simulink model "Cmd_vectorielle_simscape_tri5"  (R2018b)
settings: Solver=ode4  StartTime=0.0  StopTime=Tsim_all  FixedStep=Ts  RelTol=1e-4
values from neighbouring files (symbols this model uses):
  Clarke = [2/3 -1/3 -1/3;0 1/sqrt(3) -1/sqrt(3);1/3 1/3 1/3]    [Init_MS.m]
  Cn = Pn*rendn/Wn    (= 4.58366236105)    [Init_MS.m]
  delay_torque = 15    [Init_MS.m]
  fv = 0.0033    [Init_MS.m]
  IClarke = [1 0 1;-1/2 sqrt(3)/2 1;-1/2 -sqrt(3)/2 1]    [Init_MS.m]
  Idref = 0    [Init_MS.m]
  J = 0.05    [Init_MS.m]
  kc = 3/2*p*Phi_f    (= 2.133)    [Init_MS.m]
  Kpd_simscape = n*Rs    (= 42)    [Init_MS.m]
  Kpq_simscape = n*Rs    (= 42)    [Init_MS.m]
  kv = 5*fv/kc    (= 0.00773558368495)    [Init_MS.m]
  Ld = 0.245    [Init_MS.m]
  Lq = Ld    (= 0.245)    [Init_MS.m]
  p = 2    [Init_MS.m]
  Phi_f = 0.711    [Init_MS.m]
  r = 0.8    [Init_MS.m]
  Rs = 10.5    [Init_MS.m]
  Tid = Ld/Rs    (= 0.0233333333333)    [Init_MS.m]
  Tiq = Lq/Rs    (= 0.0233333333333)    [Init_MS.m]
  Ts = 1e-5    (= 1e-05)    [Init_MS.m]
  Vdc = 550    [Init_MS.m]
  Vn = 220    [Init_MS.m]
  Wn = Nn*2*pi/60    (= 157.079632679)    [Init_MS.m]
libraries: powerlib x5, powerlib_meascontrol x1
Description:
  | Copyright 2008-2020 The MathWorks, Inc.
settings Model: ExtModeTrigMode=oneshot  ExtModeArmWhenConnect=off  ExtModeAutoUpdateStatusClock=off  Creator=MathWorks  LastModifiedBy=jras
settings SolverCC: ZeroCrossAlgorithm=Adaptive
settings DataIOCC: ExternalInput=[]  SaveFormat=Array  SignalLoggingSaveFormat=ModelDataLogs  SaveOutput=off  SignalLogging=off  DSMLogging=off  SaveTime=off  SignalLoggingName=sigsOut
settings OptimizationCC: BlockReduction=off  BooleanDataType=off  ExpressionDepthLimit=2147483647  InitFltsAndDblsToZero=on  EfficientMapNaN2IntZero=off  LifeSpan=inf
settings DebuggingCC: UnderspecifiedInitializationDetection=Classic  MergeDetectMultiDrivingBlocksExec=none  CheckExecutionContextPreStartOutputMsg=on  CheckExecutionContextRuntimeOutputMsg=on  SignalResolutionControl=TryResolveAllWithWarning  IgnoredZcDiagnostic=none  MultiTaskDSMMsg=warning  MultiTaskCondExecSysMsg=none  SigSpecEnsureSampleTimeMsg=none  FcnCallInpInsideContextMsg=warning  StateNameClashWarn=warning  SFUnexpectedBacktrackingDiag=warning  SFNoUnconditionalDefaultTransitionDiag=warning  SFExecutionAtInitializationDiag=none
settings HardwareCC: ProdBitPerPointer=32  ProdBitPerSizeT=32  ProdBitPerPtrDiffT=32  ProdLargestAtomicFloat=None  ProdIntDivRoundTo=Undefined  ProdEndianess=Unspecified  ProdWordSize=32  ProdHWDeviceType=32-bit Generic  TargetUnknown=on
settings ModelReferenceCC: PropagateSignalLabelsOutOfModel=off
settings SFSimCC: SimUseLocalCustomCode=off
settings RTWCC: RTWUseLocalCustomCode=off
settings CodeAppCC: StateflowObjectComments=on
settings GRTTargetCC: TargetLangStandard=C89/C90 (ANSI)  GeneratePreprocessorConditionals=Disable all  CombineOutputUpdateFcns=off  GRTInterface=on
settings ConfigComp: CovMetricSettings=dw  CovHtmlReporting=on  CovSaveCumulativeToWorkspaceVar=on  CovSaveSingleToWorkspaceVar=on  CovExternalEMLEnable=off  CovSFcnEnable=off
settings SimscapeCC: SimscapeNormalizeSystem=off  SimscapeNominalValues={1, 'bar'; 1, 'cm^3/s'; 1, 'bar*kg/s'; 1, 'kJ/kg'; 1, 'kW'; }

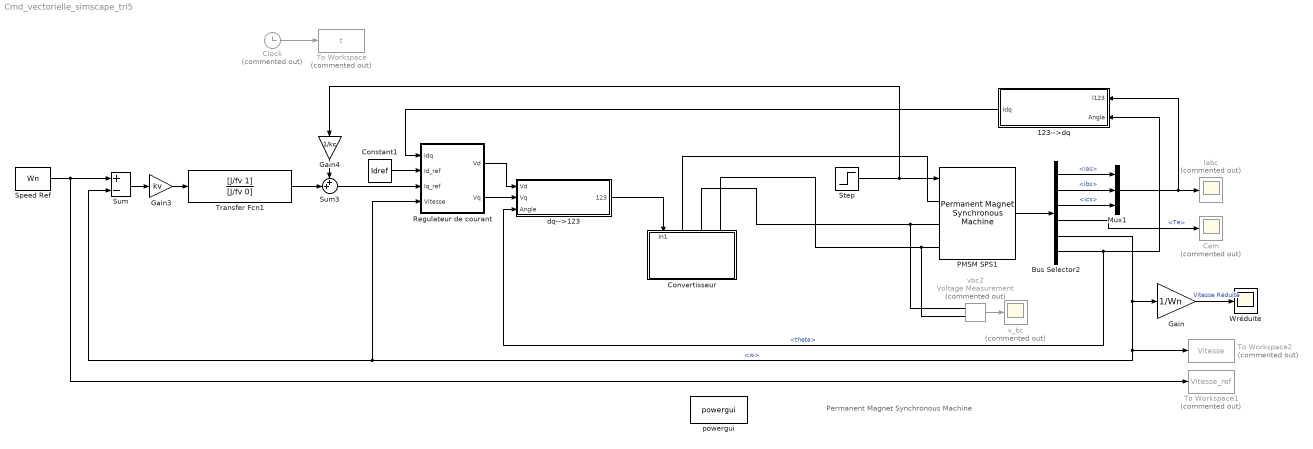
== system Cmd_vectorielle_simscape_tri5 ==
  note: Permanent Magnet Synchronous Machine
  123-->dq : Subsystem
  Bus Selector2 : BusSelector  OutputSignals=ias,ibs,ics,Te,w,theta
  Cem : Scope  Commented=on
  Clock : Clock  Commented=on
  Constant1 : Constant  Value=Idref
  Convertisseur : Subsystem
  Gain : Gain  Gain=1/Wn
  Gain3 : Gain  Gain=kv
  Gain4 : Gain  Gain=1/kc
  Iabc : Scope  Commented=on
  Mux1 : Mux  Inputs=3
  PMSM SPS1 : powerlib/Machines/Permanent Magnet Synchronous Machine  NbPhases=3  FluxDistribution=Sinusoidal  RotorType=Salient-pole  MechanicalLoad=Torque Tm  PresetModel=No  ShowDetailedParameters=on  MeasurementBus=on  Resistance=Rs  Inductance=8.5e-3  dqInductances=[Ld,Lq]  La=2*Ld  MachineConstant=Flux linkage established by magnets (V.s)  Flux=Phi_f  VoltageCst=257.9223  TorqueCst=2.133  Flat=120  Mechanical=[J fv p 0]  PolePairs=p  InitialConditions=[0,0, 0,0]  InitialConditions5ph=[0 0 0 0 0 0]  TsPowergui=0  TsBlock=-1  RefAngle=Aligned with phase A axis (original Park)
      link override From: GotoTag=T59_5719_5834794708720
  Regulateur de courant : Subsystem
  Speed Ref : Constant  Value=Wn
  Step : Step  Time=delay_torque  After=Cn  SampleTime=0
  Sum : Sum  Inputs=+-  SaturateOnIntegerOverflow=on  InputSameDT=on  OutDataTypeStr=Inherit: Same as first input
  Sum3 : Sum  Inputs=++|
  To Workspace : ToWorkspace  Commented=on  VariableName=t  SampleTime=-1
  To Workspace1 : ToWorkspace  Commented=on  VariableName=Vitesse_ref  SampleTime=-1
  To Workspace2 : ToWorkspace  Commented=on  VariableName=Vitesse  SampleTime=-1
  Transfer Fcn1 : TransferFcn  Numerator=[J/fv 1]  Denominator=[J/fv 0]
  Wréduite : Scope
  dq-->123 : Subsystem
  powergui : powerlib/powergui  SimulationMode=Discrete  SampleTime=Ts  frequency=60  Iterations=50  frequencyindice=0  Pbase=100e6  ErrMax=1e-4  UnitsV=kV  UnitsW=MW  buscounter=0  FunctionMessages=off  echomessages=off  EnableUseOfTLC=off  CurrentSourceSwitches=off  DisableSnubberDevices=off  DisableRonSwitches=off  DisableVfSwitches=off  DisplayEquations=off  SolverType=Tustin  Interpol=off  ExternalGateDelay=off  methode=off  Ts=0  x0status=blocks  SPID=on  SwTol=0  HookPort=off  RestoreLinks=warning  ResistiveCurrentMeasurement=off  Frange=[0:2:500]  Ylog=off  Xlog=on  ShowGrid=off  save=off  variable=ZData  structure=0  ZoomFFT=on  StartTime=0.0  cycles=1  DisplayStyle=1  fundamental=60  FreqAxis=off  MaxFrequency=1000  frequencyindicesteady=1  RmsSteady=1  display=off
  v_bc : Scope  Commented=on
  vbc2 : powerlib/Measurements/Voltage Measurement  Tag=PoWeRsYsTeMmEaSuReMeNt  Commented=on  PhasorSimulation=off  OutputType=Magnitude  PSBequivalent=0
      settings: SourceProductName=Simscape Electrical
  wires:
  Speed Ref/1 -> Sum/1, To Workspace1/1
  vbc2/1 -> v_bc/1
  Sum/1 -> Gain3/1
  Transfer Fcn1/1 -> Sum3/2
  Constant1/1 -> Regulateur de courant/2(Id_ref)
  Gain3/1 -> Transfer Fcn1/1
  Bus Selector2/6 -> 123-->dq/2(Angle), dq-->123/3(Angle)  "<theta>"
  Bus Selector2/2 -> Mux1/2  "<ibs>"
  Bus Selector2/1 -> Mux1/1  "<ias>"
  Bus Selector2/5 -> To Workspace2/1, Regulateur de courant/4(Vitesse), Sum/2, Gain/1  "<w>"
  Bus Selector2/3 -> Mux1/3  "<ics>"
  PMSM SPS1/1 -> Bus Selector2/1
  Mux1/1 -> Iabc/1, 123-->dq/1(I123)
  123-->dq/1(Idq) -> Regulateur de courant/1(Idq)
  Regulateur de courant/1(Vd) -> dq-->123/1(Vd)
  Regulateur de courant/2(Vq) -> dq-->123/2(Vq)
  Sum3/1 -> Regulateur de courant/3(Iq_ref)
  Gain4/1 -> Sum3/1
  Bus Selector2/4 -> Cem/1  "<Te>"
  Step/1 -> PMSM SPS1/1, Gain4/1
  Clock/1 -> To Workspace/1
  dq-->123/1(123) -> Convertisseur/1(In1)
  Gain/1 -> Wréduite/1  "Vitesse Réduite"
  connections:
  PMSM SPS1/LConn3 -- vbc2/LConn2 -- Convertisseur/LConn3
  PMSM SPS1/LConn2 -- vbc2/LConn1 -- Convertisseur/LConn2
  Convertisseur/LConn1 -- PMSM SPS1/LConn1

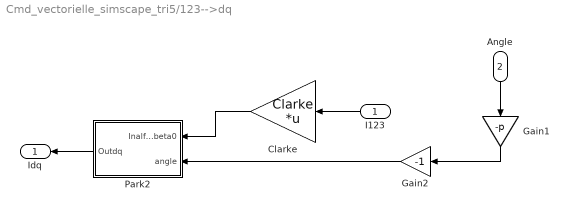
== system Cmd_vectorielle_simscape_tri5/123-->dq ==
  I123 : Inport
  Angle : Inport  Port=2
  Clarke : Gain  Gain=Clarke  Multiplication=Matrix(K*u)
  Gain1 : Gain  Gain=-p
  Gain2 : Gain  Gain=-1
  Park2 : Subsystem
  Idq : Outport
  wires:
  Angle/1 -> Gain1/1
  Gain1/1 -> Gain2/1
  Clarke/1 -> Park2/1(Inalfabeta0)
  Gain2/1 -> Park2/2(angle)
  Park2/1(Outdq) -> Idq/1
  I123/1 -> Clarke/1

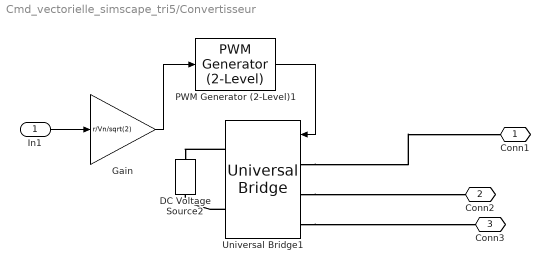
== system Cmd_vectorielle_simscape_tri5/Convertisseur ==
  In1 : Inport
  DC Voltage Source2 : powerlib/Electrical Sources/DC Voltage Source  Amplitude=Vdc  Measurements=None
      settings: SourceProductName=Simscape Electrical
  Gain : Gain  Gain=r/Vn/sqrt(2)
  PWM Generator (2-Level)1 : powerlib_meascontrol/Pulse & Signal Generators/PWM Generator (2-Level)  ModulatorType=Three-phase bridge (6 pulses)  ModulatorMode=Unsynchronized  Fc=fh  Pc=0  nF=27  MinMax="[ -1  1 ]"  SamplingTechnique=Natural  ModulatingSignals=off  m=0.8  Freq=60  Phase=0  Ts=Ts  ShowCarrierOutport=off
  Universal Bridge1 : powerlib/Power Electronics/Universal Bridge  Arms=3  SnubberResistance=1e5  SnubberCapacitance=inf  Device=IGBT / Diodes  Ron=1e-3  Lon=0  ForwardVoltages="[  0  0  ]"  ForwardVoltage=0  GTOparameters=[ 10e-6 , 20e-6 ]  IGBTparameters=[ 1e-6 , 2e-6 ]  Measurements=None  Measurements_2=None  converterType=Rectifier
      settings: SourceProductName=Simscape Electrical
  Conn1 : PMIOPort  Side=Left
  Conn2 : PMIOPort  Port=2  Side=Left
  Conn3 : PMIOPort  Port=3  Side=Left
  wires:
  Gain/1 -> PWM Generator (2-Level)1/1
  In1/1 -> Gain/1
  PWM Generator (2-Level)1/1 -> Universal Bridge1/1
  connections:
  Universal Bridge1/LConn3 -- Conn3/RConn1
  Universal Bridge1/RConn2 -- DC Voltage Source2/LConn1
  Universal Bridge1/LConn1 -- Conn1/RConn1
  Universal Bridge1/LConn2 -- Conn2/RConn1
  Universal Bridge1/RConn1 -- DC Voltage Source2/RConn1

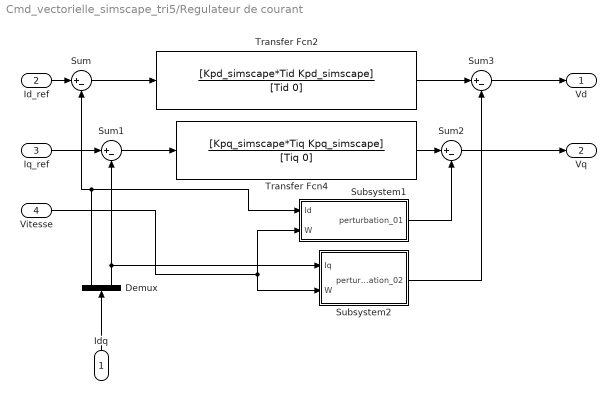
== system Cmd_vectorielle_simscape_tri5/Regulateur de courant ==
  Idq : Inport
  Id_ref : Inport  Port=2
  Iq_ref : Inport  Port=3
  Vitesse : Inport  Port=4
  Demux : Demux  Outputs=2
  Subsystem1 : Subsystem
  Subsystem2 : Subsystem
  Sum{,1..3} (4 alike) : Sum  Inputs=|+-
  Transfer Fcn2 : TransferFcn  Numerator=[Kpd_simscape*Tid Kpd_simscape]  Denominator=[Tid 0]
  Transfer Fcn4 : TransferFcn  Numerator=[Kpq_simscape*Tiq Kpq_simscape]  Denominator=[Tiq 0]
  Vd : Outport
  Vq : Outport  Port=2
  wires:
  Demux/1 -> Sum/2, Subsystem1/1(Id)
  Subsystem2/1(perturbation_02) -> Sum3/2
  Demux/2 -> Sum1/2, Subsystem2/1(Iq)
  Vitesse/1 -> Subsystem2/2(W), Subsystem1/2(W)
  Sum/1 -> Transfer Fcn2/1
  Iq_ref/1 -> Sum1/1
  Transfer Fcn4/1 -> Sum2/1
  Sum1/1 -> Transfer Fcn4/1
  Transfer Fcn2/1 -> Sum3/1
  Subsystem1/1(perturbation_01) -> Sum2/2
  Sum2/1 -> Vq/1
  Sum3/1 -> Vd/1
  Idq/1 -> Demux/1
  Id_ref/1 -> Sum/1

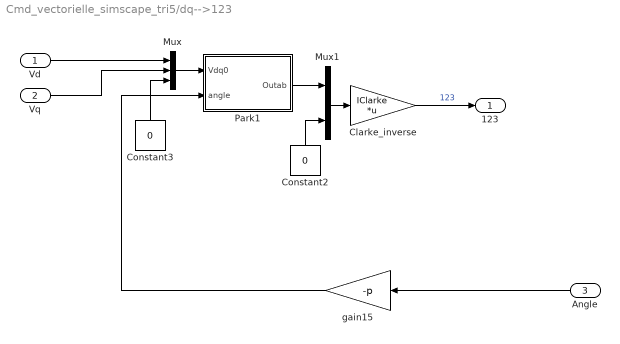
== system Cmd_vectorielle_simscape_tri5/dq-->123 ==
  Vd : Inport
  Vq : Inport  Port=2
  Angle : Inport  Port=3
  Clarke_inverse : Gain  Gain=IClarke  Multiplication=Matrix(K*u)
  Constant2 : Constant  Value=0
  Constant3 : Constant  Value=0
  Mux : Mux  Inputs=3
  Mux1 : Mux  Inputs=2
  Park1 : Subsystem
  gain15 : Gain  Gain=-p
  123 : Outport
  wires:
  Mux/1 -> Park1/1(Vdq0)
  Angle/1 -> gain15/1
  Constant2/1 -> Mux1/2
  Park1/1(Outab) -> Mux1/1
  Mux1/1 -> Clarke_inverse/1
  Vd/1 -> Mux/1
  Clarke_inverse/1 -> 123/1  "123"
  Constant3/1 -> Mux/3
  Vq/1 -> Mux/2
  gain15/1 -> Park1/2(angle)

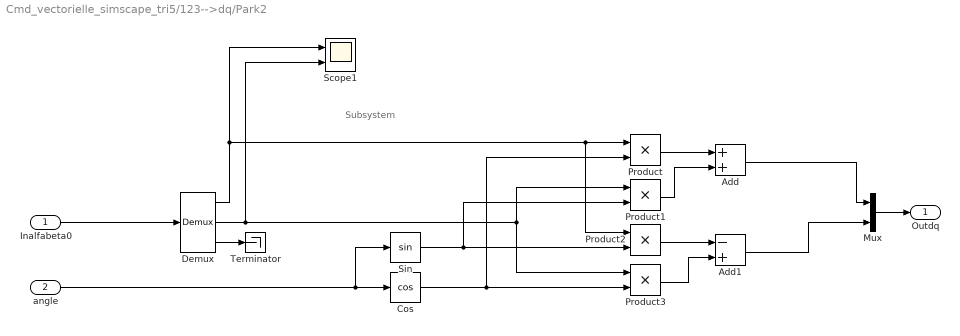
== system Cmd_vectorielle_simscape_tri5/123-->dq/Park2 ==
  note: Subsystem
  Inalfabeta0 : Inport
  angle : Inport  Port=2
  Add : Sum
  Add1 : Sum  Inputs=-+
  Cos : Trigonometry  Operator=cos
  Demux : Demux  Outputs=3
  Mux : Mux  Inputs=2
  Product{,1..3} (4 alike) : Product
  Scope1 : Scope  NumInputPorts=2
  Sin : Trigonometry
  Terminator : Terminator
  Outdq : Outport
  wires:
  Product3/1 -> Add1/2
  Product1/1 -> Add/2
  Sin/1 -> Product2/2, Product1/2
  Cos/1 -> Product3/2, Product/2
  Product/1 -> Add/1
  angle/1 -> Sin/1, Cos/1
  Demux/2 -> Product1/1, Product3/1, Scope1/2
  Demux/1 -> Scope1/1, Product2/1, Product/1
  Demux/3 -> Terminator/1
  Product2/1 -> Add1/1
  Add/1 -> Mux/1
  Add1/1 -> Mux/2
  Inalfabeta0/1 -> Demux/1
  Mux/1 -> Outdq/1

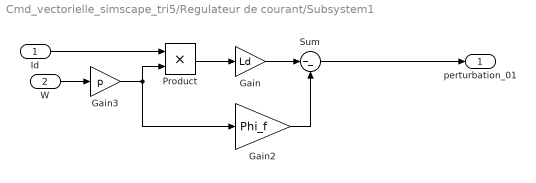
== system Cmd_vectorielle_simscape_tri5/Regulateur de courant/Subsystem1 ==
  Id : Inport
  W : Inport  Port=2
  Gain : Gain  Gain=Ld
  Gain2 : Gain  Gain=Phi_f
  Gain3 : Gain  Gain=p
  Product : Product
  Sum : Sum  Inputs=|--
  perturbation_01 : Outport
  wires:
  Id/1 -> Product/1
  Product/1 -> Gain/1
  Gain/1 -> Sum/1
  Sum/1 -> perturbation_01/1
  Gain2/1 -> Sum/2
  W/1 -> Gain3/1
  Gain3/1 -> Product/2, Gain2/1

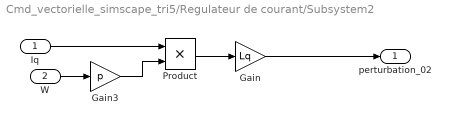
== system Cmd_vectorielle_simscape_tri5/Regulateur de courant/Subsystem2 ==
  Iq : Inport
  W : Inport  Port=2
  Gain : Gain  Gain=Lq
  Gain3 : Gain  Gain=p
  Product : Product
  perturbation_02 : Outport
  wires:
  Gain3/1 -> Product/2
  W/1 -> Gain3/1
  Gain/1 -> perturbation_02/1
  Product/1 -> Gain/1
  Iq/1 -> Product/1

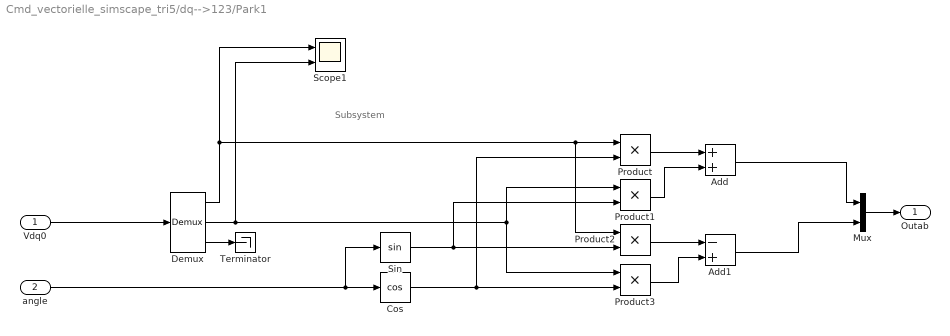
== system Cmd_vectorielle_simscape_tri5/dq-->123/Park1 ==
  note: Subsystem
  Vdq0 : Inport
  angle : Inport  Port=2
  Add : Sum
  Add1 : Sum  Inputs=-+
  Cos : Trigonometry  Operator=cos
  Demux : Demux  Outputs=3
  Mux : Mux  Inputs=2
  Product{,1..3} (4 alike) : Product
  Scope1 : Scope  NumInputPorts=2
  Sin : Trigonometry
  Terminator : Terminator
  Outab : Outport
  wires:
  Mux/1 -> Outab/1
  Vdq0/1 -> Demux/1
  Add1/1 -> Mux/2
  Add/1 -> Mux/1
  Product2/1 -> Add1/1
  Demux/3 -> Terminator/1
  Demux/1 -> Product/1, Product2/1, Scope1/1
  Demux/2 -> Scope1/2, Product3/1, Product1/1
  angle/1 -> Cos/1, Sin/1
  Product/1 -> Add/1
  Cos/1 -> Product/2, Product3/2
  Sin/1 -> Product1/2, Product2/2
  Product1/1 -> Add/2
  Product3/1 -> Add1/2
